simulink model "simulation_01"  (R2022a)
settings: Solver=VariableStepAuto  StartTime=0.0  StopTime=25  RelTol=1e-3
settings Model: Creator=Eshmith  LastModifiedBy=Eshmith

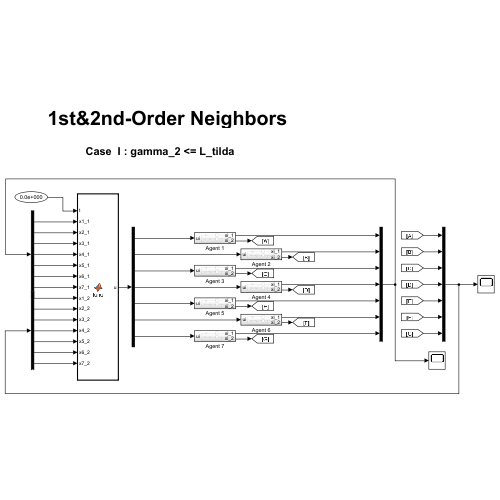
[thumbnail: Simulink's stored preview of the top-level diagram]
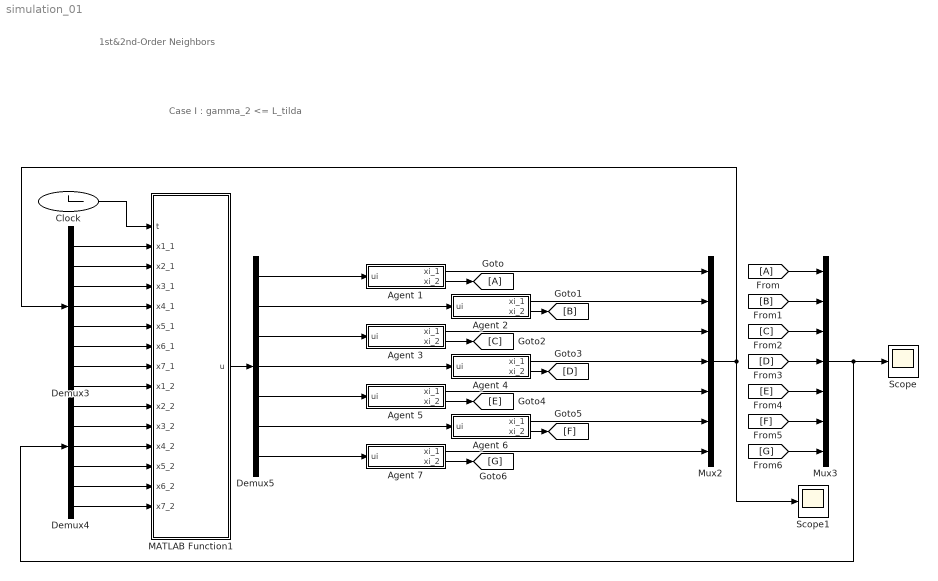
== system simulation_01 ==
  note: Case I : gamma_2 <= L_tilda
  note: 1st&2nd-Order Neighbors
  Agent 1 : Subsystem
  Agent 2 : Subsystem
  Agent 3 : Subsystem
  Agent 4 : Subsystem
  Agent 5 : Subsystem
  Agent 6 : Subsystem
  Agent 7 : Subsystem
  Clock : Clock
  Demux3 : Demux  Outputs=7
  Demux4 : Demux  Outputs=7
  Demux5 : Demux  Outputs=7
  From : From
  Goto : Goto
  MATLAB Function1 : MATLAB Function  TreatAsAtomicUnit=on
  Mux2 : Mux  Inputs=7
  Mux3 : Mux  Inputs=7
  Scope : Scope
  Scope1 : Scope
  wires:
  Demux4/1 -> MATLAB Function1/9(x1_2)
  Demux4/2 -> MATLAB Function1/10(x2_2)
  Demux4/3 -> MATLAB Function1/11(x3_2)
  Demux4/4 -> MATLAB Function1/12(x4_2)
  Demux4/5 -> MATLAB Function1/13(x5_2)
  Demux4/6 -> MATLAB Function1/14(x6_2)
  Demux4/7 -> MATLAB Function1/15(x7_2)
  Demux3/1 -> MATLAB Function1/2(x1_1)
  Demux3/2 -> MATLAB Function1/3(x2_1)
  Demux3/3 -> MATLAB Function1/4(x3_1)
  Demux3/4 -> MATLAB Function1/5(x4_1)
  Demux3/5 -> MATLAB Function1/6(x5_1)
  Demux3/6 -> MATLAB Function1/7(x6_1)
  Demux3/7 -> MATLAB Function1/8(x7_1)
  Mux3/1 -> Demux4/1, Scope/1
  Clock/1 -> MATLAB Function1/1(t)
  MATLAB Function1/1(u) -> Demux5/1
  Demux5/1 -> Agent 1/1(ui)
  Demux5/2 -> Agent 2/1(ui)
  Demux5/3 -> Agent 3/1(ui)
  Demux5/4 -> Agent 4/1(ui)
  Demux5/5 -> Agent 5/1(ui)
  Demux5/6 -> Agent 6/1(ui)
  Demux5/7 -> Agent 7/1(ui)
  Agent 1/1(xi_1) -> Mux2/1
  Agent 2/1(xi_1) -> Mux2/2
  Agent 3/1(xi_1) -> Mux2/3
  Agent 4/1(xi_1) -> Mux2/4
  Agent 5/1(xi_1) -> Mux2/5
  Agent 6/1(xi_1) -> Mux2/6
  Agent 7/1(xi_1) -> Mux2/7
  From/1 -> Mux3/1
  Agent 1/2(xi_2) -> Goto/1
  [B] -> Mux3/2
  [C] -> Mux3/3
  [D] -> Mux3/4
  [E] -> Mux3/5
  [F] -> Mux3/6
  Agent 2/2(xi_2) -> [B]
  Agent 3/2(xi_2) -> [C]
  Agent 4/2(xi_2) -> [D]
  Agent 5/2(xi_2) -> [E]
  Agent 6/2(xi_2) -> [F]
  Agent 7/2(xi_2) -> [G]
  [G] -> Mux3/7
  Mux2/1 -> Demux3/1, Scope1/1

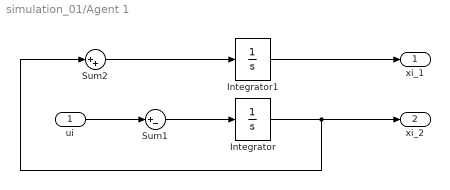
== system simulation_01/Agent 1 ==
  ui : Inport
  Integrator : Integrator  InitialCondition=-1
  Integrator1 : Integrator  InitialCondition=3.5
  Sum1 : Sum  Inputs=|+-
  Sum2 : Sum  Inputs=|++
  xi_1 : Outport
  xi_2 : Outport  Port=2
  wires:
  Sum1/1 -> Integrator/1
  ui/1 -> Sum1/1
  Integrator/1 -> Sum2/1, xi_2/1
  Integrator1/1 -> xi_1/1
  Sum2/1 -> Integrator1/1

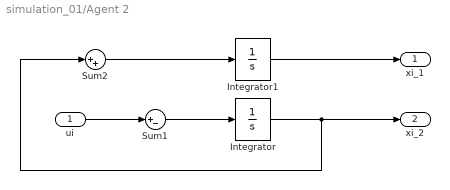
== system simulation_01/Agent 2 ==
  ui : Inport
  Integrator : Integrator  InitialCondition=-1.5
  Integrator1 : Integrator  InitialCondition=2
  Sum1 : Sum  Inputs=|+-
  Sum2 : Sum  Inputs=|++
  xi_1 : Outport
  xi_2 : Outport  Port=2
  wires:
  Sum1/1 -> Integrator/1
  ui/1 -> Sum1/1
  Integrator/1 -> Sum2/1, xi_2/1
  Integrator1/1 -> xi_1/1
  Sum2/1 -> Integrator1/1

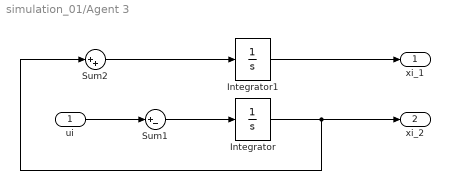
== system simulation_01/Agent 3 ==
  ui : Inport
  Integrator : Integrator  InitialCondition=-1.2
  Integrator1 : Integrator  InitialCondition=3
  Sum1 : Sum  Inputs=|+-
  Sum2 : Sum  Inputs=|++
  xi_1 : Outport
  xi_2 : Outport  Port=2
  wires:
  Sum1/1 -> Integrator/1
  ui/1 -> Sum1/1
  Integrator/1 -> Sum2/1, xi_2/1
  Integrator1/1 -> xi_1/1
  Sum2/1 -> Integrator1/1

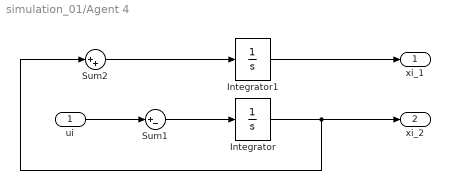
== system simulation_01/Agent 4 ==
  ui : Inport
  Integrator : Integrator  InitialCondition=1.7
  Integrator1 : Integrator  InitialCondition=3.7
  Sum1 : Sum  Inputs=|+-
  Sum2 : Sum  Inputs=|++
  xi_1 : Outport
  xi_2 : Outport  Port=2
  wires:
  Sum1/1 -> Integrator/1
  ui/1 -> Sum1/1
  Integrator/1 -> Sum2/1, xi_2/1
  Integrator1/1 -> xi_1/1
  Sum2/1 -> Integrator1/1

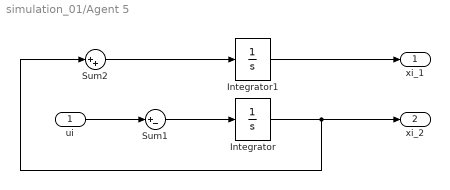
== system simulation_01/Agent 5 ==
  ui : Inport
  Integrator : Integrator  InitialCondition=1.8
  Integrator1 : Integrator  InitialCondition=2.2
  Sum1 : Sum  Inputs=|+-
  Sum2 : Sum  Inputs=|++
  xi_1 : Outport
  xi_2 : Outport  Port=2
  wires:
  Sum1/1 -> Integrator/1
  ui/1 -> Sum1/1
  Integrator/1 -> Sum2/1, xi_2/1
  Integrator1/1 -> xi_1/1
  Sum2/1 -> Integrator1/1

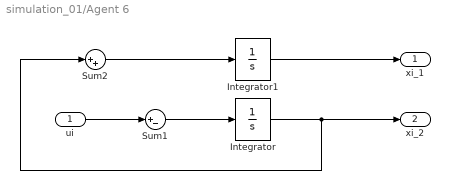
== system simulation_01/Agent 6 ==
  ui : Inport
  Integrator : Integrator  InitialCondition=1.4
  Integrator1 : Integrator  InitialCondition=3.2
  Sum1 : Sum  Inputs=|+-
  Sum2 : Sum  Inputs=|++
  xi_1 : Outport
  xi_2 : Outport  Port=2
  wires:
  Sum1/1 -> Integrator/1
  ui/1 -> Sum1/1
  Integrator/1 -> Sum2/1, xi_2/1
  Integrator1/1 -> xi_1/1
  Sum2/1 -> Integrator1/1

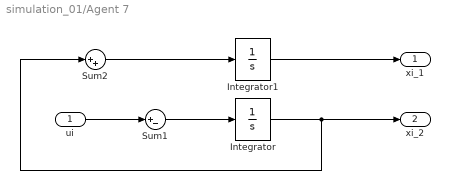
== system simulation_01/Agent 7 ==
  ui : Inport
  Integrator : Integrator  InitialCondition=1.9
  Integrator1 : Integrator  InitialCondition=3.3
  Sum1 : Sum  Inputs=|+-
  Sum2 : Sum  Inputs=|++
  xi_1 : Outport
  xi_2 : Outport  Port=2
  wires:
  Sum1/1 -> Integrator/1
  ui/1 -> Sum1/1
  Integrator/1 -> Sum2/1, xi_2/1
  Integrator1/1 -> xi_1/1
  Sum2/1 -> Integrator1/1

== matlab function simulation_01/MATLAB Function1 ==
  data: t input; x1_1 input; u output; x2_1 input; x3_1 input; x4_1 input; x5_1 input; x6_1 input; x7_1 input; x1_2 input; x2_2 input; x3_2 input; x4_2 input; x5_2 input; x6_2 input; x7_2 input
function u = func(t, x1_1, ...
                     x2_1, ...
                     x3_1, ...
                     x4_1, ...
                     x5_1, ...
                     x6_1, ...
                     x7_1, ...
                     x1_2, ...
                     x2_2, ...
                     x3_2, ...
                     x4_2, ...
                     x5_2, ...
                     x6_2, ...
                     x7_2)

states_1 = [x1_1, x2_1, x3_1, x4_1, x5_1, x6_1, x7_1, ]';
states_2 = [x1_2, x2_2, x3_2, x4_2, x5_2, x6_2, x7_2, ]';
numSates = 7;

L_1st_neighbour = [  2,-1,0,0,0,0,-1;
                     -1,2,-1,0,0,0,0;
                     0,-1,2,-1,0,0,0;
                     0,0,-1,2,-1,0,0;
                     0,0,0,-1,2,-1,0;
                     0,0,0,0,-1,2,-1;
                     -1,0,0,0,0,-1,2;];

L_tilda = [ 4 -1 -1  0  0 -1 -1;
           -1  4 -1 -1  0  0 -1;
           -1 -1  4 -1 -1  0  0;
            0 -1 -1  4 -1 -1  0;
            0  0 -1 -1  4 -1 -1;
           -1  0  0 -1 -1  4 -1;
           -1 -1  0  0 -1 -1  4;
           ];

L_2nd_neighbour = L_tilda - L_1st_neighbour;

eigLtilda = eig(L_tilda);
eigLtilda = sort(round(eigLtilda*1000)/1000);

eigL1st = eig(L_1st_neighbour);
eigL1st = sort(round(eigL1st*1000)/1000);

gamma_1 = 1;
gamma_2 = sqrt(4*gamma_1/eigLtilda(2));

u =  real(-gamma_1*L_1st_neighbour*states_1 - gamma_2*L_1st_neighbour*states_2 - gamma_1*L_2nd_neighbour*states_1 - gamma_2*L_2nd_neighbour*states_2);

end
